simulink model "imageSendExample3"  (R2014a)
settings: configuration reference "AR_Drone_ConfigSet" (kept outside this file)
libraries: AR_Drone_2_Library x3, ARdrone_video_lib x1
settings Model: SimulationMode=external  Creator=Catarina  LastModifiedBy=Catarina

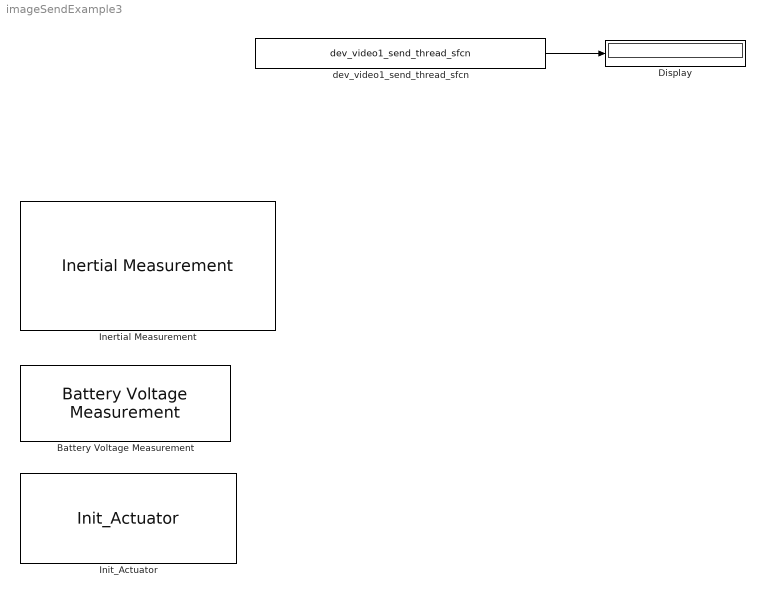
== system imageSendExample3 ==
  Battery Voltage Measurement : AR_Drone_2_Library/Battery Voltage Measurement  SFunctionSpec=void BatteryMeasure_step(single y1[1])  SampleTime=-1
  Display : Display
  Inertial Measurement : AR_Drone_2_Library/Inertial Measurement  Ts=1/400
  Init_Actuator : AR_Drone_2_Library/Init_Actuator  ShowSpec=off
  dev_video1_send_thread_sfcn : ARdrone_video_lib/dev_video1_send_thread_sfcn  SFunctionSpec=double y1 = video1GrabSendMultiThread(int32 work1[1])  SParameter1=[25300]  SParameter2=16  SParameter3=1  SampleTime=1/20  ShowSpec=on
  wires:
  dev_video1_send_thread_sfcn/1 -> Display/1
